simulink model "TP2_continu"  (R2017a)
settings: Solver=FixedStepAuto  StartTime=0.0  StopTime=30  FixedStep=0.05  RelTol=1e-3
undefined symbols (not defined in the file or in its folder): alpha0, alpha0_point
libraries: simulink x1
settings Model: Creator=rxambili  LastModifiedBy=rxambili

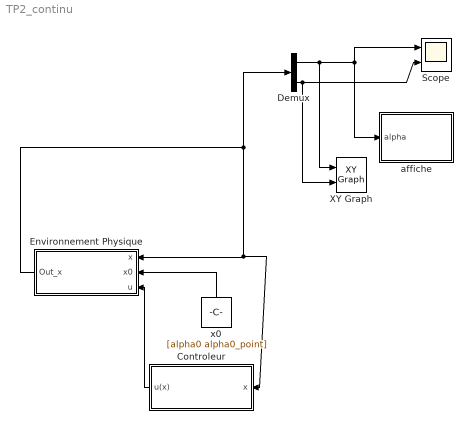
== system TP2_continu ==
  Controleur : Subsystem
  Demux : Demux  Outputs=2
  Environnement Physique : Subsystem
  Scope : Scope  NumInputPorts=2
  XY Graph : simulink/Sinks/XY Graph  xmin=-1  xmax=1  ymin=-1  ymax=1  st=-1
  "affiche " : MATLAB Function  TreatAsAtomicUnit=on
  x0 : Constant  Value=[alpha0 alpha0_point]
  wires:
  Demux/1 -> XY Graph/1, "affiche "/1(alpha), Scope/1
  Controleur/1(u(x)) -> Environnement Physique/3(u)
  x0/1 -> Environnement Physique/2(x0)
  Demux/2 -> Scope/2, XY Graph/2
  Environnement Physique/1(Out_x) -> Demux/1, Controleur/1(x), Environnement Physique/1(x)

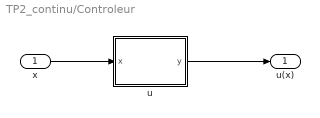
== system TP2_continu/Controleur ==
  x : Inport
  u : MATLAB Function  TreatAsAtomicUnit=on
  u(x) : Outport
  wires:
  x/1 -> u/1(x)
  u/1(y) -> u(x)/1

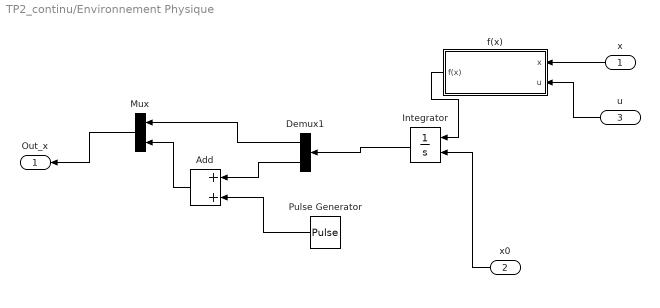
== system TP2_continu/Environnement Physique ==
  x : Inport
  x0 : Inport  Port=2
  u : Inport  Port=3
  Add : Sum
  Demux1 : Demux  Outputs=2
  Integrator : Integrator  InitialConditionSource=external  InitialCondition=[alpha0 0]
  Mux : Mux  Inputs=2
  Pulse Generator : DiscretePulseGenerator  PulseType=Time based  Amplitude=10  Period=10  PulseWidth=0.5  SampleTime=0.05
  f(x) : Subsystem
  Out_x : Outport
  wires:
  f(x)/1(f(x)) -> Integrator/1
  x0/1 -> Integrator/2
  u/1 -> f(x)/2(u)
  Add/1 -> Mux/2
  Pulse Generator/1 -> Add/2
  Demux1/2 -> Add/1
  Demux1/1 -> Mux/1
  Integrator/1 -> Demux1/1
  Mux/1 -> Out_x/1
  x/1 -> f(x)/1(x)

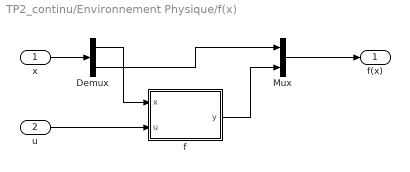
== system TP2_continu/Environnement Physique/f(x) ==
  x : Inport
  u : Inport  Port=2
  Demux : Demux  Outputs=2
  Mux : Mux  Inputs=2
  f : MATLAB Function  TreatAsAtomicUnit=on
  f(x) : Outport
  wires:
  Mux/1 -> f(x)/1
  Demux/2 -> Mux/1
  f/1(y) -> Mux/2
  u/1 -> f/2(u)
  x/1 -> Demux/1
  Demux/1 -> f/1(x)

== matlab function TP2_continu/Controleur/u ==
  data: x input; y output
function y = u(x)
u_e = 0;
K= [20 10];
x_e = [0;0];
y = u_e + K*(x-x_e);

== matlab function TP2_continu/Environnement Physique/f(x)/f ==
  data: x input; u input; y output
function y = f(x,u)
g=9.81;
l=10;
y = (g/l)*sin(x) - u*cos(x)/l;

== matlab function TP2_continu/affiche  ==
  data: alpha input
function affiche(alpha)
l=10;
x= l*sin(alpha);
y= l*cos(alpha);
figure(1);
plot([x,0],[y,0]);
axis([-1.5*l 1.5*l -1.5*l 1.5*l]);
